simulink model "Raider_walk"  (R2016a)
settings: Solver=FixedStepAuto  StartTime=0.0  StopTime=inf  FixedStep=0.01  RelTol=1e-3
model workspace (MAT data in the model file):
  SL_ROS_VariableLengthArrays_MaxSizes : struct (value not decoded)
  MCOS : class17 (value not decoded)
  MCOS : class17 (value not decoded)
libraries: robotlib x81
(part 2 of 2)

== matlab function Raider_walk/MATLAB Function ==
  data: stop output; targetPosition data_store_memory; steps input

function stop = raider_walk(steps)
% It takes as input the number of steps the robot should walk and stops the simulation when it finishes
% This controller is partially based on the Raider motion library developed by Javier Isabel, whose code is available at https://github.com/JavierIH/raider/blob/develop/code/opencm/motion/raider_motion.cpp

 setTargetPosition(0,0,0,0,0,0,0,0,0,0,0,0,0.55,0.55,-0.9625,-0.9625,0.4125,0.4125,0,0); % Initial movement. The robot at start is standing; all joints are in zero radians in this pose. The robot prepares itself for walking by bending its legs slightly to lower the global center of mass
 move(0.5);
 delay(2);
 
 
% Gait parameters 
 alpha = 0.2 % rad
 beta = 0.1 % rad 
 gamma = 0.15 % rad
 motionTime = 0.1 % seconds
 
 % During simulation it was found that a short pause between steps gives the robot more stability when walking
 stepPause = 0.04 % seconds
 
 
 
 
% Actual gait cycle. The robot always begins taking a right step
 moveVertical(0,alpha);
 moveForward(-beta, beta);
 moveShoulderSwing(-gamma,gamma);
 move(motionTime); % move up right foot and move forward right arm
 moveVertical(0,-alpha);
 move(motionTime); % move down right foot
 delay(stepPause);

 if steps > 1

     n = 2;

     while n < steps
         moveVertical(alpha,0);
         moveForward(2*beta,-2*beta);
         moveShoulderSwing(2*gamma,-2*gamma);
         move(motionTime); % move up left foot and move forward/backward left/right arm
         moveVertical(-alpha,0);
         move(motionTime); % move down left foot

         delay(stepPause);

         n = n+1;

         if n < steps

             moveVertical(0,alpha);
             moveForward(-2*beta,2*beta);
             moveShoulderSwing(-2*gamma,2*gamma);
             move(motionTime); % move up right foot and move forward/backward right/left arm
             moveVertical(0,-alpha);
             move(motionTime); % move down right foot

             delay(stepPause);

             n = n+1;
         end
     end
     
 % If the input argument "steps" is an even number the last step is done with the left foot. Else if this number is odd the last step is done with the right foot.   
     if rem(steps,2)==0        
         moveVertical(alpha,0);
         moveForward(beta,-beta);
         moveShoulderSwing(gamma,-gamma);
         move(motionTime);
         moveVertical(-alpha,0);
         move(motionTime);
     else
         moveVertical(0,alpha);
         moveForward(-beta,beta);
         moveShoulderSwing(-gamma,gamma);
         move(motionTime);
         moveVertical(0,-alpha);
         move(motionTime);            
     end


     delay(3);

     setTargetPosition(0,0,0,0,0,0,0,0,0,0,0,0,0,0,0,0,0,0,0,0); % The robot recovers the default standing position
     move(1);

 end
     
stop = true;

== matlab function Raider_walk/Simulink Function/MATLAB Function ==
  data: t input
function delay(t)

% It is used to pause “t” seconds (the time specified in move(t)) the execution of 
% the program when a movement is being done by the robot: receives as input the desired time 
% to delay the execution of the controller model, then it calls getSimTime to know the 
% current simulation time and stores this value. 
% 
% Finally, in a while-loop it compares if the elapsed time in simulation matches the 
% desired delay time, subtracting the stored value from the time returned by calling again 
% getSimTime. Since the simulation time is affected by the real-time factor, which defines 
% how much real time passes with each simulation step and this is constantly varying, 
% the elapsed time in Gazebo never coincides with the elapsed time in Simulink. 
% The Robotics System Toolbox does not provide currently any automatic solution to this issue, 
% so the delayfunction was implemented as a workaround to synchronize Simulink and Gazebo.

referenceTime = getSimTime();


while true
    currentSimTime = getSimTime();
    deltaTime= currentSimTime-referenceTime;
    if deltaTime >= t
        disp(deltaTime);
        break;
    end

end
